simulink model "PSB_FPGAdesign8_model"  (R2021a)
settings: Solver=VariableStepAuto  StartTime=0.0  StopTime=3000  RelTol=1e-3
values from neighbouring files (symbols this model uses):
  n_channel = 1024    [PSB3_0_script.m]    (also in PSB_FPGAdesign8_script.m)
  parallel_factor = 4    [PSB3_0_script.m]    (also in PSB_FPGAdesign8_script.m)
libraries: xbsIndex_r4 x1089, xrbsSSR_Library x150, dspsrcs4 x48
(part 2 of 7)

== system PSB_FPGAdesign8_model/0001_ ==
  rst : Inport
  en : Inport  Port=2
  Constant17 : xbsIndex_r4/Constant  const=3  gui_display_data_type=Fixed-point  arith_type=Unsigned  n_bits=2  bin_pt=0  preci_type=Single  exp_width=8  frac_width=24  explicit_period=on  period=1  equ=P=C  opselect=C  inp2=PCIN>>17  opr=+  inp1=P  carry=CIN  dbl_ovrd=off  block_type=constant
  Counter : xbsIndex_r4/Counter  cnt_type=Free Running  cnt_to=3  operation=Up  start_count=0  cnt_by_val=1  arith_type=Unsigned  n_bits=2  bin_pt=0  load_pin=off  rst=on  en=on  explicit_period=on  period=1  use_behavioral_HDL=off  implementation=Fabric  dbl_ovrd=off  block_type=counter
  Register : xbsIndex_r4/Register  init=0  rst=on  en=on  dbl_ovrd=off  block_type=register
  Relational : xbsIndex_r4/Relational  mode=a>=b  op_type=Bool  en=off  latency=1  dbl_ovrd=off  block_type=relational
  const : xbsIndex_r4/Constant  const=1  gui_display_data_type=Boolean  arith_type=Boolean  n_bits=18  bin_pt=16  preci_type=Single  exp_width=8  frac_width=24  explicit_period=on  period=1  equ=P=C  opselect=C  inp2=PCIN>>17  opr=+  inp1=P  carry=CIN  dbl_ovrd=off  block_type=constant
  out : Outport
  wires:
  Counter/1 -> Relational/1
  const/1 -> Register/1
  rst/1 -> Counter/1, Register/2
  Register/1 -> out/1
  Constant17/1 -> Relational/2
  Relational/1 -> Register/3
  en/1 -> Counter/2

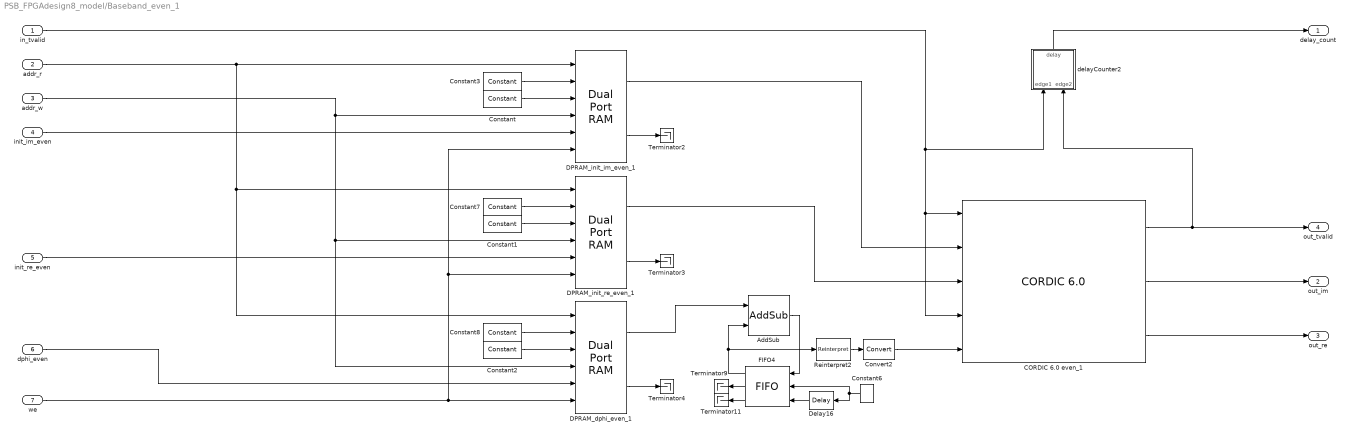
== system PSB_FPGAdesign8_model/Baseband_even_1 ==
  in_tvalid : Inport
  addr_r : Inport  Port=2
  addr_w : Inport  Port=3
  init_im_even : Inport  Port=4
  init_re_even : Inport  Port=5
  dphi_even : Inport  Port=6
  we : Inport  Port=7
  AddSub : xbsIndex_r4/AddSub  mode=Addition  use_carryin=off  use_carryout=off  en=off  latency=2  precision=User Defined  arith_type=Unsigned  n_bits=16  bin_pt=0  quantization=Truncate  overflow=Wrap  use_behavioral_HDL=off  hw_selection=Fabric  pipelined=off  dbl_ovrd=off  block_type=addsub
  "CORDIC 6.0 even_1 " : xbsIndex_r4/CORDIC 6.0   functional_selection=Rotate  architectural_configuration=Parallel  pipelining_mode=Optimal  data_format=SignedFraction  phase_format=Scaled_Radians  input_width=18  output_width=16  round_mode=Nearest_Even  iterations=16  precision=20  compensation_scaling=LUT_based  coarse_rotation=on  aclken=off  aresetn=off  out_tready=off  cartesian_has_tuser=off  cartesian_has_tlast=off  cartesian_tuser_width=1  phase_has_tuser=off  phase_has_tlast=off  phase_tuser_width=1  out_tlast_behv=Null  flow_control=NonBlocking  optimize_goal=Resources  trim_axipin_name=on  simulation_type=hybrid_sim  simulation_model=sysgen:cordic_v6_0  data_path_portlist={'s_axis_cartesian_tdata_imag', 's_axis_cartesian_tdata_real', 's_axis_phase_tdata_phase', 'm_axis_dout_tdata_imag', 'm_axis_dout_tdata_real', 'm_axis_dout_tdata_phase','m_axis_dout_tdata'}  ip_name=CORDIC  ip_version=6.0  dsptool_ready=true  ipcore_usecache=true  ipcore_useipmodelcache=true  wrapper_available=true  port_translation_map={ 'aclken' => 'en', 'aresetn' => 'rst' }  block_type=cordic_v6_0
      settings: infoedit=CORDIC 6.0
  Constant : xbsIndex_r4/Constant  const=0  gui_display_data_type=Boolean  arith_type=Boolean  n_bits=16  bin_pt=14  preci_type=Single  exp_width=8  frac_width=24  explicit_period=on  period=1  equ=P=C  opselect=C  inp2=PCIN>>17  opr=+  inp1=P  carry=CIN  dbl_ovrd=off  block_type=constant
  Constant1 : xbsIndex_r4/Constant  const=0  gui_display_data_type=Boolean  arith_type=Boolean  n_bits=16  bin_pt=14  preci_type=Single  exp_width=8  frac_width=24  explicit_period=on  period=1  equ=P=C  opselect=C  inp2=PCIN>>17  opr=+  inp1=P  carry=CIN  dbl_ovrd=off  block_type=constant
  Constant2 : xbsIndex_r4/Constant  const=0  gui_display_data_type=Boolean  arith_type=Boolean  n_bits=16  bin_pt=14  preci_type=Single  exp_width=8  frac_width=24  explicit_period=on  period=1  equ=P=C  opselect=C  inp2=PCIN>>17  opr=+  inp1=P  carry=CIN  dbl_ovrd=off  block_type=constant
  Constant3 : xbsIndex_r4/Constant  const=0  gui_display_data_type=Fixed-point  arith_type=Signed (2's comp)  n_bits=18  bin_pt=16  preci_type=Single  exp_width=8  frac_width=24  explicit_period=on  period=1  equ=P=C  opselect=C  inp2=PCIN>>17  opr=+  inp1=P  carry=CIN  dbl_ovrd=off  block_type=constant
  Constant6 : xbsIndex_r4/Constant  const=1  gui_display_data_type=Boolean  arith_type=Boolean  n_bits=16  bin_pt=14  preci_type=Single  exp_width=8  frac_width=24  explicit_period=on  period=1  equ=P=C  opselect=C  inp2=PCIN>>17  opr=+  inp1=P  carry=CIN  dbl_ovrd=off  block_type=constant
  Constant7 : xbsIndex_r4/Constant  const=0  gui_display_data_type=Fixed-point  arith_type=Signed (2's comp)  n_bits=18  bin_pt=16  preci_type=Single  exp_width=8  frac_width=24  explicit_period=on  period=1  equ=P=C  opselect=C  inp2=PCIN>>17  opr=+  inp1=P  carry=CIN  dbl_ovrd=off  block_type=constant
  Constant8 : xbsIndex_r4/Constant  const=0  gui_display_data_type=Fixed-point  arith_type=Unsigned  n_bits=16  bin_pt=0  preci_type=Single  exp_width=8  frac_width=24  explicit_period=on  period=1  equ=P=C  opselect=C  inp2=PCIN>>17  opr=+  inp1=P  carry=CIN  dbl_ovrd=off  block_type=constant
  Convert2 : xbsIndex_r4/Convert  gui_display_data_type=Fixed-point  arith_type="Signed  (2's comp)"  n_bits=18  bin_pt=15  float_type=Single  exp_bits=8  fraction_bits=24  quantization=Truncate  overflow=Wrap  en=off  latency=0  pipeline=off  dbl_ovrd=off  block_type=convert
  DPRAM_dphi_even_1 : xbsIndex_r4/Dual Port RAM  depth=n_channel/parallel_factor  initVector=dphi_uint16_even_1  distributed_mem=Block RAM  init_a=0  init_b=0  rst_a=off  rst_b=off  en_a=off  en_b=off  latency=1  write_mode_A=Read Before Write  write_mode_B=Read Before Write  optimize=Area  dbl_ovrd=off  simulation_type=fast_sim  block_type=dpram
  DPRAM_init_im_even_1 : xbsIndex_r4/Dual Port RAM  depth=n_channel/parallel_factor  initVector=init_im_even_1  distributed_mem=Block RAM  init_a=0  init_b=0  rst_a=off  rst_b=off  en_a=off  en_b=off  latency=1  write_mode_A=Read Before Write  write_mode_B=Read Before Write  optimize=Area  dbl_ovrd=off  simulation_type=fast_sim  block_type=dpram
  DPRAM_init_re_even_1 : xbsIndex_r4/Dual Port RAM  depth=n_channel/parallel_factor  initVector=init_re_even_1  distributed_mem=Block RAM  init_a=0  init_b=0  rst_a=off  rst_b=off  en_a=off  en_b=off  latency=1  write_mode_A=Read Before Write  write_mode_B=Read Before Write  optimize=Area  dbl_ovrd=off  simulation_type=fast_sim  block_type=dpram
  Delay16 : xbsIndex_r4/Delay  rst=off  infoeditControl=Selection of Reset will increase slice count due to use of real FFs and instead of SRLs  en=off  latency=n_channel/parallel_factor-2-1  reg_retiming=off  dbl_ovrd=off  block_type=delay
  FIFO4 : xbsIndex_r4/FIFO  mem_type=Block RAM  performance_options=Standard_FIFO  embedded_registers=off  depth=1K  percent_nbits=1  rst=off  rst_latency=2  en=off  use_dcount=off  use_percent_full_port=off  use_almost_empty=off  almost_empty_thresh=2  use_almost_full=off  use_rd_rst_busy=off  use_wr_rst_busy=off  almost_full_thresh=14  explicit_period=off  dbl_ovrd=off  simulation_type=fast_sim  block_type=fifo
  Reinterpret2 : xbsIndex_r4/Reinterpret  force_arith_type=on  arith_type="Signed  (2's comp)"  force_bin_pt=on  bin_pt=15  block_type=reinterpret
  Terminator{2..4,9,11} (5 alike) : Terminator
  delayCounter2 : Subsystem
  delay_count : Outport
  out_im : Outport  Port=2
  out_re : Outport  Port=3
  out_tvalid : Outport  Port=4
  wires:
  in_tvalid/1 -> "CORDIC 6.0 even_1 "/1, "CORDIC 6.0 even_1 "/4, delayCounter2/1(edge1)
  "CORDIC 6.0 even_1 "/1 -> out_tvalid/1, delayCounter2/2(edge2)
  Reinterpret2/1 -> Convert2/1
  FIFO4/2 -> Terminator9/1
  dphi_even/1 -> DPRAM_dphi_even_1/5
  delayCounter2/1(delay) -> delay_count/1
  Constant1/1 -> DPRAM_init_re_even_1/3
  FIFO4/3 -> Terminator11/1
  Constant2/1 -> DPRAM_dphi_even_1/3
  Constant3/1 -> DPRAM_init_im_even_1/2
  addr_w/1 -> DPRAM_init_im_even_1/4, DPRAM_init_re_even_1/4, DPRAM_dphi_even_1/4
  Constant6/1 -> Delay16/1, FIFO4/2
  Convert2/1 -> "CORDIC 6.0 even_1 "/5
  Constant7/1 -> DPRAM_init_re_even_1/2
  DPRAM_dphi_even_1/2 -> Terminator4/1
  Delay16/1 -> FIFO4/3
  FIFO4/1 -> Reinterpret2/1, AddSub/2
  init_im_even/1 -> DPRAM_init_im_even_1/5
  we/1 -> DPRAM_init_im_even_1/6, DPRAM_init_re_even_1/6, DPRAM_dphi_even_1/6
  addr_r/1 -> DPRAM_init_im_even_1/1, DPRAM_init_re_even_1/1, DPRAM_dphi_even_1/1
  DPRAM_init_re_even_1/2 -> Terminator3/1
  Constant8/1 -> DPRAM_dphi_even_1/2
  DPRAM_init_im_even_1/1 -> "CORDIC 6.0 even_1 "/2
  DPRAM_init_re_even_1/1 -> "CORDIC 6.0 even_1 "/3
  DPRAM_dphi_even_1/1 -> AddSub/1
  DPRAM_init_im_even_1/2 -> Terminator2/1
  "CORDIC 6.0 even_1 "/3 -> out_re/1
  Constant/1 -> DPRAM_init_im_even_1/3
  AddSub/1 -> FIFO4/1
  init_re_even/1 -> DPRAM_init_re_even_1/5
  "CORDIC 6.0 even_1 "/2 -> out_im/1

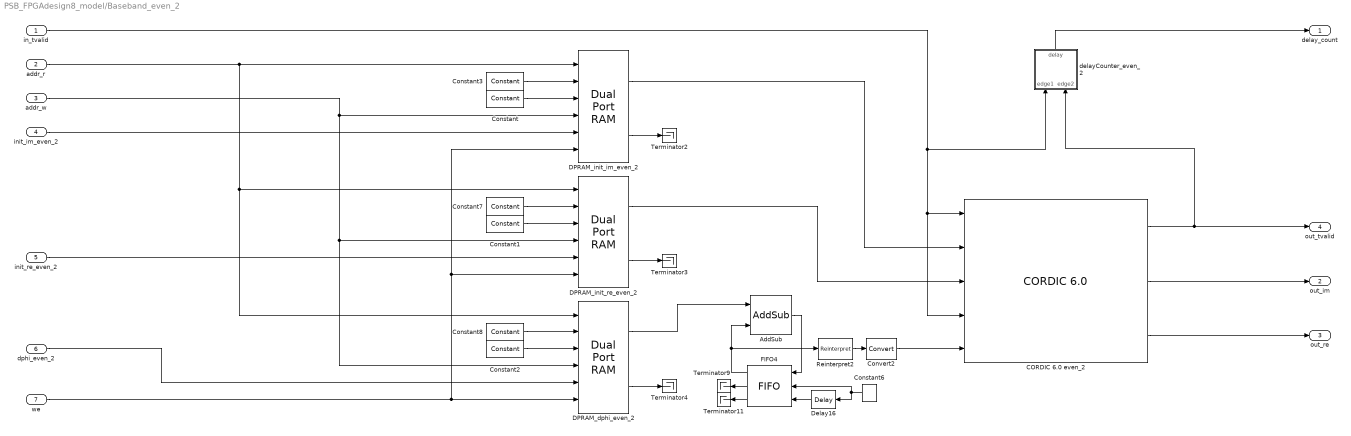
== system PSB_FPGAdesign8_model/Baseband_even_2 ==
  in_tvalid : Inport
  addr_r : Inport  Port=2
  addr_w : Inport  Port=3
  init_im_even_2 : Inport  Port=4
  init_re_even_2 : Inport  Port=5
  dphi_even_2 : Inport  Port=6
  we : Inport  Port=7
  AddSub : xbsIndex_r4/AddSub  mode=Addition  use_carryin=off  use_carryout=off  en=off  latency=2  precision=User Defined  arith_type=Unsigned  n_bits=16  bin_pt=0  quantization=Truncate  overflow=Wrap  use_behavioral_HDL=off  hw_selection=Fabric  pipelined=off  dbl_ovrd=off  block_type=addsub
  CORDIC 6.0 even_2 : xbsIndex_r4/CORDIC 6.0   functional_selection=Rotate  architectural_configuration=Parallel  pipelining_mode=Optimal  data_format=SignedFraction  phase_format=Scaled_Radians  input_width=18  output_width=16  round_mode=Nearest_Even  iterations=16  precision=20  compensation_scaling=LUT_based  coarse_rotation=on  aclken=off  aresetn=off  out_tready=off  cartesian_has_tuser=off  cartesian_has_tlast=off  cartesian_tuser_width=1  phase_has_tuser=off  phase_has_tlast=off  phase_tuser_width=1  out_tlast_behv=Null  flow_control=NonBlocking  optimize_goal=Resources  trim_axipin_name=on  simulation_type=hybrid_sim  simulation_model=sysgen:cordic_v6_0  data_path_portlist={'s_axis_cartesian_tdata_imag', 's_axis_cartesian_tdata_real', 's_axis_phase_tdata_phase', 'm_axis_dout_tdata_imag', 'm_axis_dout_tdata_real', 'm_axis_dout_tdata_phase','m_axis_dout_tdata'}  ip_name=CORDIC  ip_version=6.0  dsptool_ready=true  ipcore_usecache=true  ipcore_useipmodelcache=true  wrapper_available=true  port_translation_map={ 'aclken' => 'en', 'aresetn' => 'rst' }  block_type=cordic_v6_0
      settings: infoedit=CORDIC 6.0
  Constant : xbsIndex_r4/Constant  const=0  gui_display_data_type=Boolean  arith_type=Boolean  n_bits=16  bin_pt=14  preci_type=Single  exp_width=8  frac_width=24  explicit_period=on  period=1  equ=P=C  opselect=C  inp2=PCIN>>17  opr=+  inp1=P  carry=CIN  dbl_ovrd=off  block_type=constant
  Constant1 : xbsIndex_r4/Constant  const=0  gui_display_data_type=Boolean  arith_type=Boolean  n_bits=16  bin_pt=14  preci_type=Single  exp_width=8  frac_width=24  explicit_period=on  period=1  equ=P=C  opselect=C  inp2=PCIN>>17  opr=+  inp1=P  carry=CIN  dbl_ovrd=off  block_type=constant
  Constant2 : xbsIndex_r4/Constant  const=0  gui_display_data_type=Boolean  arith_type=Boolean  n_bits=16  bin_pt=14  preci_type=Single  exp_width=8  frac_width=24  explicit_period=on  period=1  equ=P=C  opselect=C  inp2=PCIN>>17  opr=+  inp1=P  carry=CIN  dbl_ovrd=off  block_type=constant
  Constant3 : xbsIndex_r4/Constant  const=0  gui_display_data_type=Fixed-point  arith_type=Signed (2's comp)  n_bits=18  bin_pt=16  preci_type=Single  exp_width=8  frac_width=24  explicit_period=on  period=1  equ=P=C  opselect=C  inp2=PCIN>>17  opr=+  inp1=P  carry=CIN  dbl_ovrd=off  block_type=constant
  Constant6 : xbsIndex_r4/Constant  const=1  gui_display_data_type=Boolean  arith_type=Boolean  n_bits=16  bin_pt=14  preci_type=Single  exp_width=8  frac_width=24  explicit_period=on  period=1  equ=P=C  opselect=C  inp2=PCIN>>17  opr=+  inp1=P  carry=CIN  dbl_ovrd=off  block_type=constant
  Constant7 : xbsIndex_r4/Constant  const=0  gui_display_data_type=Fixed-point  arith_type=Signed (2's comp)  n_bits=18  bin_pt=16  preci_type=Single  exp_width=8  frac_width=24  explicit_period=on  period=1  equ=P=C  opselect=C  inp2=PCIN>>17  opr=+  inp1=P  carry=CIN  dbl_ovrd=off  block_type=constant
  Constant8 : xbsIndex_r4/Constant  const=0  gui_display_data_type=Fixed-point  arith_type=Unsigned  n_bits=16  bin_pt=0  preci_type=Single  exp_width=8  frac_width=24  explicit_period=on  period=1  equ=P=C  opselect=C  inp2=PCIN>>17  opr=+  inp1=P  carry=CIN  dbl_ovrd=off  block_type=constant
  Convert2 : xbsIndex_r4/Convert  gui_display_data_type=Fixed-point  arith_type="Signed  (2's comp)"  n_bits=18  bin_pt=15  float_type=Single  exp_bits=8  fraction_bits=24  quantization=Truncate  overflow=Wrap  en=off  latency=0  pipeline=off  dbl_ovrd=off  block_type=convert
  DPRAM_dphi_even_2 : xbsIndex_r4/Dual Port RAM  depth=n_channel/parallel_factor  initVector=dphi_uint16_even_2  distributed_mem=Block RAM  init_a=0  init_b=0  rst_a=off  rst_b=off  en_a=off  en_b=off  latency=1  write_mode_A=Read Before Write  write_mode_B=Read Before Write  optimize=Area  dbl_ovrd=off  simulation_type=fast_sim  block_type=dpram
  DPRAM_init_im_even_2 : xbsIndex_r4/Dual Port RAM  depth=n_channel/parallel_factor  initVector=init_im_even_2  distributed_mem=Block RAM  init_a=0  init_b=0  rst_a=off  rst_b=off  en_a=off  en_b=off  latency=1  write_mode_A=Read Before Write  write_mode_B=Read Before Write  optimize=Area  dbl_ovrd=off  simulation_type=fast_sim  block_type=dpram
  DPRAM_init_re_even_2 : xbsIndex_r4/Dual Port RAM  depth=n_channel/parallel_factor  initVector=init_re_even_2  distributed_mem=Block RAM  init_a=0  init_b=0  rst_a=off  rst_b=off  en_a=off  en_b=off  latency=1  write_mode_A=Read Before Write  write_mode_B=Read Before Write  optimize=Area  dbl_ovrd=off  simulation_type=fast_sim  block_type=dpram
  Delay16 : xbsIndex_r4/Delay  rst=off  infoeditControl=Selection of Reset will increase slice count due to use of real FFs and instead of SRLs  en=off  latency=n_channel/parallel_factor-2-1  reg_retiming=off  dbl_ovrd=off  block_type=delay
  FIFO4 : xbsIndex_r4/FIFO  mem_type=Block RAM  performance_options=Standard_FIFO  embedded_registers=off  depth=1K  percent_nbits=1  rst=off  rst_latency=2  en=off  use_dcount=off  use_percent_full_port=off  use_almost_empty=off  almost_empty_thresh=2  use_almost_full=off  use_rd_rst_busy=off  use_wr_rst_busy=off  almost_full_thresh=14  explicit_period=off  dbl_ovrd=off  simulation_type=fast_sim  block_type=fifo
  Reinterpret2 : xbsIndex_r4/Reinterpret  force_arith_type=on  arith_type="Signed  (2's comp)"  force_bin_pt=on  bin_pt=15  block_type=reinterpret
  Terminator{2..4,9,11} (5 alike) : Terminator
  delayCounter_even_2 : Subsystem
  delay_count : Outport
  out_im : Outport  Port=2
  out_re : Outport  Port=3
  out_tvalid : Outport  Port=4
  wires:
  CORDIC 6.0 even_2/2 -> out_im/1
  init_re_even_2/1 -> DPRAM_init_re_even_2/5
  AddSub/1 -> FIFO4/1
  Constant/1 -> DPRAM_init_im_even_2/3
  CORDIC 6.0 even_2/3 -> out_re/1
  DPRAM_init_im_even_2/2 -> Terminator2/1
  DPRAM_dphi_even_2/1 -> AddSub/1
  DPRAM_init_re_even_2/1 -> CORDIC 6.0 even_2/3
  DPRAM_init_im_even_2/1 -> CORDIC 6.0 even_2/2
  Constant8/1 -> DPRAM_dphi_even_2/2
  DPRAM_init_re_even_2/2 -> Terminator3/1
  addr_r/1 -> DPRAM_dphi_even_2/1, DPRAM_init_re_even_2/1, DPRAM_init_im_even_2/1
  we/1 -> DPRAM_dphi_even_2/6, DPRAM_init_re_even_2/6, DPRAM_init_im_even_2/6
  init_im_even_2/1 -> DPRAM_init_im_even_2/5
  FIFO4/1 -> AddSub/2, Reinterpret2/1
  Delay16/1 -> FIFO4/3
  DPRAM_dphi_even_2/2 -> Terminator4/1
  Constant7/1 -> DPRAM_init_re_even_2/2
  Convert2/1 -> CORDIC 6.0 even_2/5
  Constant6/1 -> FIFO4/2, Delay16/1
  addr_w/1 -> DPRAM_dphi_even_2/4, DPRAM_init_re_even_2/4, DPRAM_init_im_even_2/4
  Constant3/1 -> DPRAM_init_im_even_2/2
  Constant2/1 -> DPRAM_dphi_even_2/3
  FIFO4/3 -> Terminator11/1
  Constant1/1 -> DPRAM_init_re_even_2/3
  delayCounter_even_2/1(delay) -> delay_count/1
  dphi_even_2/1 -> DPRAM_dphi_even_2/5
  FIFO4/2 -> Terminator9/1
  Reinterpret2/1 -> Convert2/1
  in_tvalid/1 -> delayCounter_even_2/1(edge1), CORDIC 6.0 even_2/4, CORDIC 6.0 even_2/1
  CORDIC 6.0 even_2/1 -> delayCounter_even_2/2(edge2), out_tvalid/1

== system PSB_FPGAdesign8_model/Baseband_even_3 ==
  in_tvalid : Inport
  addr_r : Inport  Port=2
  addr_w : Inport  Port=3
  init_im_even : Inport  Port=4
  init_re_even : Inport  Port=5
  dphi_even : Inport  Port=6
  we : Inport  Port=7
  AddSub : xbsIndex_r4/AddSub  mode=Addition  use_carryin=off  use_carryout=off  en=off  latency=2  precision=User Defined  arith_type=Unsigned  n_bits=16  bin_pt=0  quantization=Truncate  overflow=Wrap  use_behavioral_HDL=off  hw_selection=Fabric  pipelined=off  dbl_ovrd=off  block_type=addsub
  "CORDIC 6.0 even_1 " : xbsIndex_r4/CORDIC 6.0   functional_selection=Rotate  architectural_configuration=Parallel  pipelining_mode=Optimal  data_format=SignedFraction  phase_format=Scaled_Radians  input_width=18  output_width=16  round_mode=Nearest_Even  iterations=16  precision=20  compensation_scaling=LUT_based  coarse_rotation=on  aclken=off  aresetn=off  out_tready=off  cartesian_has_tuser=off  cartesian_has_tlast=off  cartesian_tuser_width=1  phase_has_tuser=off  phase_has_tlast=off  phase_tuser_width=1  out_tlast_behv=Null  flow_control=NonBlocking  optimize_goal=Resources  trim_axipin_name=on  simulation_type=hybrid_sim  simulation_model=sysgen:cordic_v6_0  data_path_portlist={'s_axis_cartesian_tdata_imag', 's_axis_cartesian_tdata_real', 's_axis_phase_tdata_phase', 'm_axis_dout_tdata_imag', 'm_axis_dout_tdata_real', 'm_axis_dout_tdata_phase','m_axis_dout_tdata'}  ip_name=CORDIC  ip_version=6.0  dsptool_ready=true  ipcore_usecache=true  ipcore_useipmodelcache=true  wrapper_available=true  port_translation_map={ 'aclken' => 'en', 'aresetn' => 'rst' }  block_type=cordic_v6_0
      settings: infoedit=CORDIC 6.0
  Constant : xbsIndex_r4/Constant  const=0  gui_display_data_type=Boolean  arith_type=Boolean  n_bits=16  bin_pt=14  preci_type=Single  exp_width=8  frac_width=24  explicit_period=on  period=1  equ=P=C  opselect=C  inp2=PCIN>>17  opr=+  inp1=P  carry=CIN  dbl_ovrd=off  block_type=constant
  Constant1 : xbsIndex_r4/Constant  const=0  gui_display_data_type=Boolean  arith_type=Boolean  n_bits=16  bin_pt=14  preci_type=Single  exp_width=8  frac_width=24  explicit_period=on  period=1  equ=P=C  opselect=C  inp2=PCIN>>17  opr=+  inp1=P  carry=CIN  dbl_ovrd=off  block_type=constant
  Constant2 : xbsIndex_r4/Constant  const=0  gui_display_data_type=Boolean  arith_type=Boolean  n_bits=16  bin_pt=14  preci_type=Single  exp_width=8  frac_width=24  explicit_period=on  period=1  equ=P=C  opselect=C  inp2=PCIN>>17  opr=+  inp1=P  carry=CIN  dbl_ovrd=off  block_type=constant
  Constant3 : xbsIndex_r4/Constant  const=0  gui_display_data_type=Fixed-point  arith_type=Signed (2's comp)  n_bits=18  bin_pt=16  preci_type=Single  exp_width=8  frac_width=24  explicit_period=on  period=1  equ=P=C  opselect=C  inp2=PCIN>>17  opr=+  inp1=P  carry=CIN  dbl_ovrd=off  block_type=constant
  Constant6 : xbsIndex_r4/Constant  const=1  gui_display_data_type=Boolean  arith_type=Boolean  n_bits=16  bin_pt=14  preci_type=Single  exp_width=8  frac_width=24  explicit_period=on  period=1  equ=P=C  opselect=C  inp2=PCIN>>17  opr=+  inp1=P  carry=CIN  dbl_ovrd=off  block_type=constant
  Constant7 : xbsIndex_r4/Constant  const=0  gui_display_data_type=Fixed-point  arith_type=Signed (2's comp)  n_bits=18  bin_pt=16  preci_type=Single  exp_width=8  frac_width=24  explicit_period=on  period=1  equ=P=C  opselect=C  inp2=PCIN>>17  opr=+  inp1=P  carry=CIN  dbl_ovrd=off  block_type=constant
  Constant8 : xbsIndex_r4/Constant  const=0  gui_display_data_type=Fixed-point  arith_type=Unsigned  n_bits=16  bin_pt=0  preci_type=Single  exp_width=8  frac_width=24  explicit_period=on  period=1  equ=P=C  opselect=C  inp2=PCIN>>17  opr=+  inp1=P  carry=CIN  dbl_ovrd=off  block_type=constant
  Convert2 : xbsIndex_r4/Convert  gui_display_data_type=Fixed-point  arith_type="Signed  (2's comp)"  n_bits=18  bin_pt=15  float_type=Single  exp_bits=8  fraction_bits=24  quantization=Truncate  overflow=Wrap  en=off  latency=0  pipeline=off  dbl_ovrd=off  block_type=convert
  DPRAM_dphi_even_3 : xbsIndex_r4/Dual Port RAM  depth=n_channel/parallel_factor  initVector=dphi_uint16_even_3  distributed_mem=Block RAM  init_a=0  init_b=0  rst_a=off  rst_b=off  en_a=off  en_b=off  latency=1  write_mode_A=Read Before Write  write_mode_B=Read Before Write  optimize=Area  dbl_ovrd=off  simulation_type=fast_sim  block_type=dpram
  DPRAM_init_im_even_3 : xbsIndex_r4/Dual Port RAM  depth=n_channel/parallel_factor  initVector=init_im_even_3  distributed_mem=Block RAM  init_a=0  init_b=0  rst_a=off  rst_b=off  en_a=off  en_b=off  latency=1  write_mode_A=Read Before Write  write_mode_B=Read Before Write  optimize=Area  dbl_ovrd=off  simulation_type=fast_sim  block_type=dpram
  DPRAM_init_re_even_3 : xbsIndex_r4/Dual Port RAM  depth=n_channel/parallel_factor  initVector=init_re_even_3  distributed_mem=Block RAM  init_a=0  init_b=0  rst_a=off  rst_b=off  en_a=off  en_b=off  latency=1  write_mode_A=Read Before Write  write_mode_B=Read Before Write  optimize=Area  dbl_ovrd=off  simulation_type=fast_sim  block_type=dpram
  Delay16 : xbsIndex_r4/Delay  rst=off  infoeditControl=Selection of Reset will increase slice count due to use of real FFs and instead of SRLs  en=off  latency=n_channel/parallel_factor-2-1  reg_retiming=off  dbl_ovrd=off  block_type=delay
  FIFO4 : xbsIndex_r4/FIFO  mem_type=Block RAM  performance_options=Standard_FIFO  embedded_registers=off  depth=1K  percent_nbits=1  rst=off  rst_latency=2  en=off  use_dcount=off  use_percent_full_port=off  use_almost_empty=off  almost_empty_thresh=2  use_almost_full=off  use_rd_rst_busy=off  use_wr_rst_busy=off  almost_full_thresh=14  explicit_period=off  dbl_ovrd=off  simulation_type=fast_sim  block_type=fifo
  Reinterpret2 : xbsIndex_r4/Reinterpret  force_arith_type=on  arith_type="Signed  (2's comp)"  force_bin_pt=on  bin_pt=15  block_type=reinterpret
  Terminator{2..4,9,11} (5 alike) : Terminator
  delayCounter2 : Subsystem
  delay_count : Outport
  out_im : Outport  Port=2
  out_re : Outport  Port=3
  out_tvalid : Outport  Port=4
  wires:
  "CORDIC 6.0 even_1 "/2 -> out_im/1
  init_re_even/1 -> DPRAM_init_re_even_3/5
  AddSub/1 -> FIFO4/1
  Constant/1 -> DPRAM_init_im_even_3/3
  "CORDIC 6.0 even_1 "/3 -> out_re/1
  DPRAM_init_im_even_3/2 -> Terminator2/1
  DPRAM_dphi_even_3/1 -> AddSub/1
  DPRAM_init_re_even_3/1 -> "CORDIC 6.0 even_1 "/3
  DPRAM_init_im_even_3/1 -> "CORDIC 6.0 even_1 "/2
  Constant8/1 -> DPRAM_dphi_even_3/2
  DPRAM_init_re_even_3/2 -> Terminator3/1
  addr_r/1 -> DPRAM_dphi_even_3/1, DPRAM_init_re_even_3/1, DPRAM_init_im_even_3/1
  we/1 -> DPRAM_dphi_even_3/6, DPRAM_init_re_even_3/6, DPRAM_init_im_even_3/6
  init_im_even/1 -> DPRAM_init_im_even_3/5
  FIFO4/1 -> AddSub/2, Reinterpret2/1
  Delay16/1 -> FIFO4/3
  DPRAM_dphi_even_3/2 -> Terminator4/1
  Constant7/1 -> DPRAM_init_re_even_3/2
  Convert2/1 -> "CORDIC 6.0 even_1 "/5
  Constant6/1 -> FIFO4/2, Delay16/1
  addr_w/1 -> DPRAM_dphi_even_3/4, DPRAM_init_re_even_3/4, DPRAM_init_im_even_3/4
  Constant3/1 -> DPRAM_init_im_even_3/2
  Constant2/1 -> DPRAM_dphi_even_3/3
  FIFO4/3 -> Terminator11/1
  Constant1/1 -> DPRAM_init_re_even_3/3
  delayCounter2/1(delay) -> delay_count/1
  dphi_even/1 -> DPRAM_dphi_even_3/5
  FIFO4/2 -> Terminator9/1
  Reinterpret2/1 -> Convert2/1
  "CORDIC 6.0 even_1 "/1 -> delayCounter2/2(edge2), out_tvalid/1
  in_tvalid/1 -> delayCounter2/1(edge1), "CORDIC 6.0 even_1 "/4, "CORDIC 6.0 even_1 "/1

== system PSB_FPGAdesign8_model/Baseband_even_4 ==
  in_tvalid : Inport
  addr_r : Inport  Port=2
  addr_w : Inport  Port=3
  init_im_even_2 : Inport  Port=4
  init_re_even_2 : Inport  Port=5
  dphi_even_2 : Inport  Port=6
  we : Inport  Port=7
  AddSub : xbsIndex_r4/AddSub  mode=Addition  use_carryin=off  use_carryout=off  en=off  latency=2  precision=User Defined  arith_type=Unsigned  n_bits=16  bin_pt=0  quantization=Truncate  overflow=Wrap  use_behavioral_HDL=off  hw_selection=Fabric  pipelined=off  dbl_ovrd=off  block_type=addsub
  CORDIC 6.0 even_2 : xbsIndex_r4/CORDIC 6.0   functional_selection=Rotate  architectural_configuration=Parallel  pipelining_mode=Optimal  data_format=SignedFraction  phase_format=Scaled_Radians  input_width=18  output_width=16  round_mode=Nearest_Even  iterations=16  precision=20  compensation_scaling=LUT_based  coarse_rotation=on  aclken=off  aresetn=off  out_tready=off  cartesian_has_tuser=off  cartesian_has_tlast=off  cartesian_tuser_width=1  phase_has_tuser=off  phase_has_tlast=off  phase_tuser_width=1  out_tlast_behv=Null  flow_control=NonBlocking  optimize_goal=Resources  trim_axipin_name=on  simulation_type=hybrid_sim  simulation_model=sysgen:cordic_v6_0  data_path_portlist={'s_axis_cartesian_tdata_imag', 's_axis_cartesian_tdata_real', 's_axis_phase_tdata_phase', 'm_axis_dout_tdata_imag', 'm_axis_dout_tdata_real', 'm_axis_dout_tdata_phase','m_axis_dout_tdata'}  ip_name=CORDIC  ip_version=6.0  dsptool_ready=true  ipcore_usecache=true  ipcore_useipmodelcache=true  wrapper_available=true  port_translation_map={ 'aclken' => 'en', 'aresetn' => 'rst' }  block_type=cordic_v6_0
      settings: infoedit=CORDIC 6.0
  Constant : xbsIndex_r4/Constant  const=0  gui_display_data_type=Boolean  arith_type=Boolean  n_bits=16  bin_pt=14  preci_type=Single  exp_width=8  frac_width=24  explicit_period=on  period=1  equ=P=C  opselect=C  inp2=PCIN>>17  opr=+  inp1=P  carry=CIN  dbl_ovrd=off  block_type=constant
  Constant1 : xbsIndex_r4/Constant  const=0  gui_display_data_type=Boolean  arith_type=Boolean  n_bits=16  bin_pt=14  preci_type=Single  exp_width=8  frac_width=24  explicit_period=on  period=1  equ=P=C  opselect=C  inp2=PCIN>>17  opr=+  inp1=P  carry=CIN  dbl_ovrd=off  block_type=constant
  Constant2 : xbsIndex_r4/Constant  const=0  gui_display_data_type=Boolean  arith_type=Boolean  n_bits=16  bin_pt=14  preci_type=Single  exp_width=8  frac_width=24  explicit_period=on  period=1  equ=P=C  opselect=C  inp2=PCIN>>17  opr=+  inp1=P  carry=CIN  dbl_ovrd=off  block_type=constant
  Constant3 : xbsIndex_r4/Constant  const=0  gui_display_data_type=Fixed-point  arith_type=Signed (2's comp)  n_bits=18  bin_pt=16  preci_type=Single  exp_width=8  frac_width=24  explicit_period=on  period=1  equ=P=C  opselect=C  inp2=PCIN>>17  opr=+  inp1=P  carry=CIN  dbl_ovrd=off  block_type=constant
  Constant6 : xbsIndex_r4/Constant  const=1  gui_display_data_type=Boolean  arith_type=Boolean  n_bits=16  bin_pt=14  preci_type=Single  exp_width=8  frac_width=24  explicit_period=on  period=1  equ=P=C  opselect=C  inp2=PCIN>>17  opr=+  inp1=P  carry=CIN  dbl_ovrd=off  block_type=constant
  Constant7 : xbsIndex_r4/Constant  const=0  gui_display_data_type=Fixed-point  arith_type=Signed (2's comp)  n_bits=18  bin_pt=16  preci_type=Single  exp_width=8  frac_width=24  explicit_period=on  period=1  equ=P=C  opselect=C  inp2=PCIN>>17  opr=+  inp1=P  carry=CIN  dbl_ovrd=off  block_type=constant
  Constant8 : xbsIndex_r4/Constant  const=0  gui_display_data_type=Fixed-point  arith_type=Unsigned  n_bits=16  bin_pt=0  preci_type=Single  exp_width=8  frac_width=24  explicit_period=on  period=1  equ=P=C  opselect=C  inp2=PCIN>>17  opr=+  inp1=P  carry=CIN  dbl_ovrd=off  block_type=constant
  Convert2 : xbsIndex_r4/Convert  gui_display_data_type=Fixed-point  arith_type="Signed  (2's comp)"  n_bits=18  bin_pt=15  float_type=Single  exp_bits=8  fraction_bits=24  quantization=Truncate  overflow=Wrap  en=off  latency=0  pipeline=off  dbl_ovrd=off  block_type=convert
  DPRAM_dphi_even_4 : xbsIndex_r4/Dual Port RAM  depth=n_channel/parallel_factor  initVector=dphi_uint16_even_4  distributed_mem=Block RAM  init_a=0  init_b=0  rst_a=off  rst_b=off  en_a=off  en_b=off  latency=1  write_mode_A=Read Before Write  write_mode_B=Read Before Write  optimize=Area  dbl_ovrd=off  simulation_type=fast_sim  block_type=dpram
  DPRAM_init_im_even_4 : xbsIndex_r4/Dual Port RAM  depth=n_channel/parallel_factor  initVector=init_im_even_4  distributed_mem=Block RAM  init_a=0  init_b=0  rst_a=off  rst_b=off  en_a=off  en_b=off  latency=1  write_mode_A=Read Before Write  write_mode_B=Read Before Write  optimize=Area  dbl_ovrd=off  simulation_type=fast_sim  block_type=dpram
  DPRAM_init_re_even_4 : xbsIndex_r4/Dual Port RAM  depth=n_channel/parallel_factor  initVector=init_re_even_4  distributed_mem=Block RAM  init_a=0  init_b=0  rst_a=off  rst_b=off  en_a=off  en_b=off  latency=1  write_mode_A=Read Before Write  write_mode_B=Read Before Write  optimize=Area  dbl_ovrd=off  simulation_type=fast_sim  block_type=dpram
  Delay16 : xbsIndex_r4/Delay  rst=off  infoeditControl=Selection of Reset will increase slice count due to use of real FFs and instead of SRLs  en=off  latency=n_channel/parallel_factor-2-1  reg_retiming=off  dbl_ovrd=off  block_type=delay
  FIFO4 : xbsIndex_r4/FIFO  mem_type=Block RAM  performance_options=Standard_FIFO  embedded_registers=off  depth=1K  percent_nbits=1  rst=off  rst_latency=2  en=off  use_dcount=off  use_percent_full_port=off  use_almost_empty=off  almost_empty_thresh=2  use_almost_full=off  use_rd_rst_busy=off  use_wr_rst_busy=off  almost_full_thresh=14  explicit_period=off  dbl_ovrd=off  simulation_type=fast_sim  block_type=fifo
  Reinterpret2 : xbsIndex_r4/Reinterpret  force_arith_type=on  arith_type="Signed  (2's comp)"  force_bin_pt=on  bin_pt=15  block_type=reinterpret
  Terminator{2..4,9,11} (5 alike) : Terminator
  delayCounter_even_2 : Subsystem
  delay_count : Outport
  out_im : Outport  Port=2
  out_re : Outport  Port=3
  out_tvalid : Outport  Port=4
  wires:
  CORDIC 6.0 even_2/1 -> out_tvalid/1, delayCounter_even_2/2(edge2)
  in_tvalid/1 -> CORDIC 6.0 even_2/1, CORDIC 6.0 even_2/4, delayCounter_even_2/1(edge1)
  Reinterpret2/1 -> Convert2/1
  FIFO4/2 -> Terminator9/1
  dphi_even_2/1 -> DPRAM_dphi_even_4/5
  delayCounter_even_2/1(delay) -> delay_count/1
  Constant1/1 -> DPRAM_init_re_even_4/3
  FIFO4/3 -> Terminator11/1
  Constant2/1 -> DPRAM_dphi_even_4/3
  Constant3/1 -> DPRAM_init_im_even_4/2
  addr_w/1 -> DPRAM_init_im_even_4/4, DPRAM_init_re_even_4/4, DPRAM_dphi_even_4/4
  Constant6/1 -> Delay16/1, FIFO4/2
  Convert2/1 -> CORDIC 6.0 even_2/5
  Constant7/1 -> DPRAM_init_re_even_4/2
  DPRAM_dphi_even_4/2 -> Terminator4/1
  Delay16/1 -> FIFO4/3
  FIFO4/1 -> Reinterpret2/1, AddSub/2
  init_im_even_2/1 -> DPRAM_init_im_even_4/5
  we/1 -> DPRAM_init_im_even_4/6, DPRAM_init_re_even_4/6, DPRAM_dphi_even_4/6
  addr_r/1 -> DPRAM_init_im_even_4/1, DPRAM_init_re_even_4/1, DPRAM_dphi_even_4/1
  DPRAM_init_re_even_4/2 -> Terminator3/1
  Constant8/1 -> DPRAM_dphi_even_4/2
  DPRAM_init_im_even_4/1 -> CORDIC 6.0 even_2/2
  DPRAM_init_re_even_4/1 -> CORDIC 6.0 even_2/3
  DPRAM_dphi_even_4/1 -> AddSub/1
  DPRAM_init_im_even_4/2 -> Terminator2/1
  CORDIC 6.0 even_2/3 -> out_re/1
  Constant/1 -> DPRAM_init_im_even_4/3
  AddSub/1 -> FIFO4/1
  init_re_even_2/1 -> DPRAM_init_re_even_4/5
  CORDIC 6.0 even_2/2 -> out_im/1

== system PSB_FPGAdesign8_model/Baseband_odd_1 ==
  tvalid : Inport
  addr_r : Inport  Port=2
  addr_w : Inport  Port=3
  init_im_odd : Inport  Port=4
  init_re_odd : Inport  Port=5
  dphi_odd : Inport  Port=6
  we : Inport  Port=7
  AddSub1 : xbsIndex_r4/AddSub  mode=Addition  use_carryin=off  use_carryout=off  en=off  latency=2  precision=User Defined  arith_type=Unsigned  n_bits=16  bin_pt=0  quantization=Truncate  overflow=Wrap  use_behavioral_HDL=off  hw_selection=Fabric  pipelined=off  dbl_ovrd=off  block_type=addsub
  CORDIC 6.0 odd_1 : xbsIndex_r4/CORDIC 6.0   functional_selection=Rotate  architectural_configuration=Parallel  pipelining_mode=Optimal  data_format=SignedFraction  phase_format=Scaled_Radians  input_width=18  output_width=16  round_mode=Nearest_Even  iterations=16  precision=20  compensation_scaling=LUT_based  coarse_rotation=on  aclken=off  aresetn=off  out_tready=off  cartesian_has_tuser=off  cartesian_has_tlast=off  cartesian_tuser_width=1  phase_has_tuser=off  phase_has_tlast=off  phase_tuser_width=1  out_tlast_behv=Null  flow_control=NonBlocking  optimize_goal=Resources  trim_axipin_name=on  simulation_type=hybrid_sim  simulation_model=sysgen:cordic_v6_0  data_path_portlist={'s_axis_cartesian_tdata_imag', 's_axis_cartesian_tdata_real', 's_axis_phase_tdata_phase', 'm_axis_dout_tdata_imag', 'm_axis_dout_tdata_real', 'm_axis_dout_tdata_phase','m_axis_dout_tdata'}  ip_name=CORDIC  ip_version=6.0  dsptool_ready=true  ipcore_usecache=true  ipcore_useipmodelcache=true  wrapper_available=true  port_translation_map={ 'aclken' => 'en', 'aresetn' => 'rst' }  block_type=cordic_v6_0
      settings: infoedit=CORDIC 6.0
  Constant10 : xbsIndex_r4/Constant  const=0  gui_display_data_type=Fixed-point  arith_type=Signed (2's comp)  n_bits=18  bin_pt=16  preci_type=Single  exp_width=8  frac_width=24  explicit_period=on  period=1  equ=P=C  opselect=C  inp2=PCIN>>17  opr=+  inp1=P  carry=CIN  dbl_ovrd=off  block_type=constant
  Constant11 : xbsIndex_r4/Constant  const=1  gui_display_data_type=Boolean  arith_type=Boolean  n_bits=16  bin_pt=14  preci_type=Single  exp_width=8  frac_width=24  explicit_period=on  period=1  equ=P=C  opselect=C  inp2=PCIN>>17  opr=+  inp1=P  carry=CIN  dbl_ovrd=off  block_type=constant
  Constant12 : xbsIndex_r4/Constant  const=0  gui_display_data_type=Fixed-point  arith_type=Signed (2's comp)  n_bits=18  bin_pt=16  preci_type=Single  exp_width=8  frac_width=24  explicit_period=on  period=1  equ=P=C  opselect=C  inp2=PCIN>>17  opr=+  inp1=P  carry=CIN  dbl_ovrd=off  block_type=constant
  Constant13 : xbsIndex_r4/Constant  const=0  gui_display_data_type=Fixed-point  arith_type=Unsigned  n_bits=16  bin_pt=0  preci_type=Single  exp_width=8  frac_width=24  explicit_period=on  period=1  equ=P=C  opselect=C  inp2=PCIN>>17  opr=+  inp1=P  carry=CIN  dbl_ovrd=off  block_type=constant
  Constant4 : xbsIndex_r4/Constant  const=0  gui_display_data_type=Boolean  arith_type=Boolean  n_bits=16  bin_pt=14  preci_type=Single  exp_width=8  frac_width=24  explicit_period=on  period=1  equ=P=C  opselect=C  inp2=PCIN>>17  opr=+  inp1=P  carry=CIN  dbl_ovrd=off  block_type=constant
  Constant5 : xbsIndex_r4/Constant  const=0  gui_display_data_type=Boolean  arith_type=Boolean  n_bits=16  bin_pt=14  preci_type=Single  exp_width=8  frac_width=24  explicit_period=on  period=1  equ=P=C  opselect=C  inp2=PCIN>>17  opr=+  inp1=P  carry=CIN  dbl_ovrd=off  block_type=constant
  Constant9 : xbsIndex_r4/Constant  const=0  gui_display_data_type=Boolean  arith_type=Boolean  n_bits=16  bin_pt=14  preci_type=Single  exp_width=8  frac_width=24  explicit_period=on  period=1  equ=P=C  opselect=C  inp2=PCIN>>17  opr=+  inp1=P  carry=CIN  dbl_ovrd=off  block_type=constant
  Convert1 : xbsIndex_r4/Convert  gui_display_data_type=Fixed-point  arith_type="Signed  (2's comp)"  n_bits=18  bin_pt=15  float_type=Single  exp_bits=8  fraction_bits=24  quantization=Truncate  overflow=Wrap  en=off  latency=0  pipeline=off  dbl_ovrd=off  block_type=convert
  DPRAM_dphi_odd_1 : xbsIndex_r4/Dual Port RAM  depth=n_channel/parallel_factor  initVector=dphi_uint16_odd_1  distributed_mem=Block RAM  init_a=0  init_b=0  rst_a=off  rst_b=off  en_a=off  en_b=off  latency=1  write_mode_A=Read Before Write  write_mode_B=Read Before Write  optimize=Area  dbl_ovrd=off  simulation_type=fast_sim  block_type=dpram
  DPRAM_init_im_odd_1 : xbsIndex_r4/Dual Port RAM  depth=n_channel/parallel_factor  initVector=init_im_odd_1  distributed_mem=Block RAM  init_a=0  init_b=0  rst_a=off  rst_b=off  en_a=off  en_b=off  latency=1  write_mode_A=Read Before Write  write_mode_B=Read Before Write  optimize=Area  dbl_ovrd=off  simulation_type=fast_sim  block_type=dpram
  DPRAM_init_re_odd_1 : xbsIndex_r4/Dual Port RAM  depth=n_channel/parallel_factor  initVector=init_re_odd_1  distributed_mem=Block RAM  init_a=0  init_b=0  rst_a=off  rst_b=off  en_a=off  en_b=off  latency=1  write_mode_A=Read Before Write  write_mode_B=Read Before Write  optimize=Area  dbl_ovrd=off  simulation_type=fast_sim  block_type=dpram
  Delay8 : xbsIndex_r4/Delay  rst=off  infoeditControl=Selection of Reset will increase slice count due to use of real FFs and instead of SRLs  en=off  latency=n_channel/parallel_factor-2-1  reg_retiming=off  dbl_ovrd=off  block_type=delay
  FIFO1 : xbsIndex_r4/FIFO  mem_type=Block RAM  performance_options=Standard_FIFO  embedded_registers=off  depth=1K  percent_nbits=1  rst=off  rst_latency=2  en=off  use_dcount=off  use_percent_full_port=off  use_almost_empty=off  almost_empty_thresh=2  use_almost_full=off  use_rd_rst_busy=off  use_wr_rst_busy=off  almost_full_thresh=14  explicit_period=off  dbl_ovrd=off  simulation_type=fast_sim  block_type=fifo
  Reinterpret1 : xbsIndex_r4/Reinterpret  force_arith_type=on  arith_type="Signed  (2's comp)"  force_bin_pt=on  bin_pt=15  block_type=reinterpret
  Terminator{6..8,10,12} (5 alike) : Terminator
  delayCounter1 : Subsystem
  delay_count : Outport
  out_im : Outport  Port=2
  out_re : Outport  Port=3
  out_tvalid : Outport  Port=4
  wires:
  Delay8/1 -> FIFO1/3
  tvalid/1 -> CORDIC 6.0 odd_1/1, CORDIC 6.0 odd_1/4, delayCounter1/1(edge1)
  we/1 -> DPRAM_init_im_odd_1/6, DPRAM_init_re_odd_1/6, DPRAM_dphi_odd_1/6
  Constant12/1 -> DPRAM_init_re_odd_1/2
  init_re_odd/1 -> DPRAM_init_re_odd_1/5
  addr_r/1 -> DPRAM_init_im_odd_1/1, DPRAM_init_re_odd_1/1, DPRAM_dphi_odd_1/1
  FIFO1/3 -> Terminator6/1
  Constant13/1 -> DPRAM_dphi_odd_1/2
  DPRAM_init_im_odd_1/1 -> CORDIC 6.0 odd_1/2
  DPRAM_dphi_odd_1/2 -> Terminator10/1
  CORDIC 6.0 odd_1/3 -> out_re/1
  FIFO1/1 -> Reinterpret1/1, AddSub1/2
  Constant10/1 -> DPRAM_init_im_odd_1/2
  Constant5/1 -> DPRAM_init_re_odd_1/3
  Constant4/1 -> DPRAM_init_im_odd_1/3
  DPRAM_init_re_odd_1/1 -> CORDIC 6.0 odd_1/3
  Constant11/1 -> Delay8/1, FIFO1/2
  DPRAM_init_re_odd_1/2 -> Terminator8/1
  DPRAM_init_im_odd_1/2 -> Terminator7/1
  Convert1/1 -> CORDIC 6.0 odd_1/5
  AddSub1/1 -> FIFO1/1
  addr_w/1 -> DPRAM_init_im_odd_1/4, DPRAM_init_re_odd_1/4, DPRAM_dphi_odd_1/4
  Constant9/1 -> DPRAM_dphi_odd_1/3
  delayCounter1/1(delay) -> delay_count/1
  DPRAM_dphi_odd_1/1 -> AddSub1/1
  Reinterpret1/1 -> Convert1/1
  FIFO1/2 -> Terminator12/1
  dphi_odd/1 -> DPRAM_dphi_odd_1/5
  init_im_odd/1 -> DPRAM_init_im_odd_1/5
  CORDIC 6.0 odd_1/2 -> out_im/1
  CORDIC 6.0 odd_1/1 -> delayCounter1/2(edge2), out_tvalid/1

== system PSB_FPGAdesign8_model/Baseband_odd_2 ==
  tvalid : Inport
  addr_r : Inport  Port=2
  addr_w : Inport  Port=3
  init_im_odd_2 : Inport  Port=4
  init_re_odd_2 : Inport  Port=5
  dphi_odd_2 : Inport  Port=6
  we : Inport  Port=7
  AddSub1 : xbsIndex_r4/AddSub  mode=Addition  use_carryin=off  use_carryout=off  en=off  latency=2  precision=User Defined  arith_type=Unsigned  n_bits=16  bin_pt=0  quantization=Truncate  overflow=Wrap  use_behavioral_HDL=off  hw_selection=Fabric  pipelined=off  dbl_ovrd=off  block_type=addsub
  CORDIC 6.0 odd_2 : xbsIndex_r4/CORDIC 6.0   functional_selection=Rotate  architectural_configuration=Parallel  pipelining_mode=Optimal  data_format=SignedFraction  phase_format=Scaled_Radians  input_width=18  output_width=16  round_mode=Nearest_Even  iterations=16  precision=20  compensation_scaling=LUT_based  coarse_rotation=on  aclken=off  aresetn=off  out_tready=off  cartesian_has_tuser=off  cartesian_has_tlast=off  cartesian_tuser_width=1  phase_has_tuser=off  phase_has_tlast=off  phase_tuser_width=1  out_tlast_behv=Null  flow_control=NonBlocking  optimize_goal=Resources  trim_axipin_name=on  simulation_type=hybrid_sim  simulation_model=sysgen:cordic_v6_0  data_path_portlist={'s_axis_cartesian_tdata_imag', 's_axis_cartesian_tdata_real', 's_axis_phase_tdata_phase', 'm_axis_dout_tdata_imag', 'm_axis_dout_tdata_real', 'm_axis_dout_tdata_phase','m_axis_dout_tdata'}  ip_name=CORDIC  ip_version=6.0  dsptool_ready=true  ipcore_usecache=true  ipcore_useipmodelcache=true  wrapper_available=true  port_translation_map={ 'aclken' => 'en', 'aresetn' => 'rst' }  block_type=cordic_v6_0
      settings: infoedit=CORDIC 6.0
  Constant10 : xbsIndex_r4/Constant  const=0  gui_display_data_type=Fixed-point  arith_type=Signed (2's comp)  n_bits=18  bin_pt=16  preci_type=Single  exp_width=8  frac_width=24  explicit_period=on  period=1  equ=P=C  opselect=C  inp2=PCIN>>17  opr=+  inp1=P  carry=CIN  dbl_ovrd=off  block_type=constant
  Constant11 : xbsIndex_r4/Constant  const=1  gui_display_data_type=Boolean  arith_type=Boolean  n_bits=16  bin_pt=14  preci_type=Single  exp_width=8  frac_width=24  explicit_period=on  period=1  equ=P=C  opselect=C  inp2=PCIN>>17  opr=+  inp1=P  carry=CIN  dbl_ovrd=off  block_type=constant
  Constant12 : xbsIndex_r4/Constant  const=0  gui_display_data_type=Fixed-point  arith_type=Signed (2's comp)  n_bits=18  bin_pt=16  preci_type=Single  exp_width=8  frac_width=24  explicit_period=on  period=1  equ=P=C  opselect=C  inp2=PCIN>>17  opr=+  inp1=P  carry=CIN  dbl_ovrd=off  block_type=constant
  Constant13 : xbsIndex_r4/Constant  const=0  gui_display_data_type=Fixed-point  arith_type=Unsigned  n_bits=16  bin_pt=0  preci_type=Single  exp_width=8  frac_width=24  explicit_period=on  period=1  equ=P=C  opselect=C  inp2=PCIN>>17  opr=+  inp1=P  carry=CIN  dbl_ovrd=off  block_type=constant
  Constant4 : xbsIndex_r4/Constant  const=0  gui_display_data_type=Boolean  arith_type=Boolean  n_bits=16  bin_pt=14  preci_type=Single  exp_width=8  frac_width=24  explicit_period=on  period=1  equ=P=C  opselect=C  inp2=PCIN>>17  opr=+  inp1=P  carry=CIN  dbl_ovrd=off  block_type=constant
  Constant5 : xbsIndex_r4/Constant  const=0  gui_display_data_type=Boolean  arith_type=Boolean  n_bits=16  bin_pt=14  preci_type=Single  exp_width=8  frac_width=24  explicit_period=on  period=1  equ=P=C  opselect=C  inp2=PCIN>>17  opr=+  inp1=P  carry=CIN  dbl_ovrd=off  block_type=constant
  Constant9 : xbsIndex_r4/Constant  const=0  gui_display_data_type=Boolean  arith_type=Boolean  n_bits=16  bin_pt=14  preci_type=Single  exp_width=8  frac_width=24  explicit_period=on  period=1  equ=P=C  opselect=C  inp2=PCIN>>17  opr=+  inp1=P  carry=CIN  dbl_ovrd=off  block_type=constant
  Convert1 : xbsIndex_r4/Convert  gui_display_data_type=Fixed-point  arith_type="Signed  (2's comp)"  n_bits=18  bin_pt=15  float_type=Single  exp_bits=8  fraction_bits=24  quantization=Truncate  overflow=Wrap  en=off  latency=0  pipeline=off  dbl_ovrd=off  block_type=convert
  DPRAM_dphi_odd_2 : xbsIndex_r4/Dual Port RAM  depth=n_channel/parallel_factor  initVector=dphi_uint16_odd_2  distributed_mem=Block RAM  init_a=0  init_b=0  rst_a=off  rst_b=off  en_a=off  en_b=off  latency=1  write_mode_A=Read Before Write  write_mode_B=Read Before Write  optimize=Area  dbl_ovrd=off  simulation_type=fast_sim  block_type=dpram
  DPRAM_init_im_odd_2 : xbsIndex_r4/Dual Port RAM  depth=n_channel/parallel_factor  initVector=init_im_odd_2  distributed_mem=Block RAM  init_a=0  init_b=0  rst_a=off  rst_b=off  en_a=off  en_b=off  latency=1  write_mode_A=Read Before Write  write_mode_B=Read Before Write  optimize=Area  dbl_ovrd=off  simulation_type=fast_sim  block_type=dpram
  DPRAM_init_re_odd_2 : xbsIndex_r4/Dual Port RAM  depth=n_channel/parallel_factor  initVector=init_re_odd_2  distributed_mem=Block RAM  init_a=0  init_b=0  rst_a=off  rst_b=off  en_a=off  en_b=off  latency=1  write_mode_A=Read Before Write  write_mode_B=Read Before Write  optimize=Area  dbl_ovrd=off  simulation_type=fast_sim  block_type=dpram
  Delay8 : xbsIndex_r4/Delay  rst=off  infoeditControl=Selection of Reset will increase slice count due to use of real FFs and instead of SRLs  en=off  latency=n_channel/parallel_factor-2-1  reg_retiming=off  dbl_ovrd=off  block_type=delay
  FIFO1 : xbsIndex_r4/FIFO  mem_type=Block RAM  performance_options=Standard_FIFO  embedded_registers=off  depth=1K  percent_nbits=1  rst=off  rst_latency=2  en=off  use_dcount=off  use_percent_full_port=off  use_almost_empty=off  almost_empty_thresh=2  use_almost_full=off  use_rd_rst_busy=off  use_wr_rst_busy=off  almost_full_thresh=14  explicit_period=off  dbl_ovrd=off  simulation_type=fast_sim  block_type=fifo
  Reinterpret1 : xbsIndex_r4/Reinterpret  force_arith_type=on  arith_type="Signed  (2's comp)"  force_bin_pt=on  bin_pt=15  block_type=reinterpret
  Terminator{6..8,10,12} (5 alike) : Terminator
  delayCounter_odd_2 : Subsystem
  delay_count : Outport
  out_im : Outport  Port=2
  out_re : Outport  Port=3
  out_tvalid : Outport  Port=4
  wires:
  CORDIC 6.0 odd_2/2 -> out_im/1
  init_im_odd_2/1 -> DPRAM_init_im_odd_2/5
  dphi_odd_2/1 -> DPRAM_dphi_odd_2/5
  FIFO1/2 -> Terminator12/1
  Reinterpret1/1 -> Convert1/1
  DPRAM_dphi_odd_2/1 -> AddSub1/1
  delayCounter_odd_2/1(delay) -> delay_count/1
  Constant9/1 -> DPRAM_dphi_odd_2/3
  addr_w/1 -> DPRAM_dphi_odd_2/4, DPRAM_init_re_odd_2/4, DPRAM_init_im_odd_2/4
  AddSub1/1 -> FIFO1/1
  Convert1/1 -> CORDIC 6.0 odd_2/5
  DPRAM_init_im_odd_2/2 -> Terminator7/1
  DPRAM_init_re_odd_2/2 -> Terminator8/1
  Constant11/1 -> FIFO1/2, Delay8/1
  DPRAM_init_re_odd_2/1 -> CORDIC 6.0 odd_2/3
  Constant4/1 -> DPRAM_init_im_odd_2/3
  Constant5/1 -> DPRAM_init_re_odd_2/3
  Constant10/1 -> DPRAM_init_im_odd_2/2
  FIFO1/1 -> AddSub1/2, Reinterpret1/1
  CORDIC 6.0 odd_2/3 -> out_re/1
  DPRAM_dphi_odd_2/2 -> Terminator10/1
  DPRAM_init_im_odd_2/1 -> CORDIC 6.0 odd_2/2
  Constant13/1 -> DPRAM_dphi_odd_2/2
  FIFO1/3 -> Terminator6/1
  addr_r/1 -> DPRAM_dphi_odd_2/1, DPRAM_init_re_odd_2/1, DPRAM_init_im_odd_2/1
  init_re_odd_2/1 -> DPRAM_init_re_odd_2/5
  Constant12/1 -> DPRAM_init_re_odd_2/2
  we/1 -> DPRAM_dphi_odd_2/6, DPRAM_init_re_odd_2/6, DPRAM_init_im_odd_2/6
  tvalid/1 -> delayCounter_odd_2/1(edge1), CORDIC 6.0 odd_2/4, CORDIC 6.0 odd_2/1
  Delay8/1 -> FIFO1/3
  CORDIC 6.0 odd_2/1 -> delayCounter_odd_2/2(edge2), out_tvalid/1
